simulink model "FINAL_MODEL"  (R2021a)
settings: Solver=VariableStepAuto  StartTime=0.0  StopTime=100  MaxStep=1e-4  RelTol=1e-3
libraries: spsDiodeLib x6, spsIGBTLib x6, spsSeriesRLCBranchLib x3, spsVoltageMeasurementLib x3, spsAsynchronousMachineSIUnitsLib x1, spsDCVoltageSourceLib x1, spsMeanLib x1, pid_lib x1, spspowerguiLib x1
settings Model: Creator=shashank  LastModifiedBy=shashank

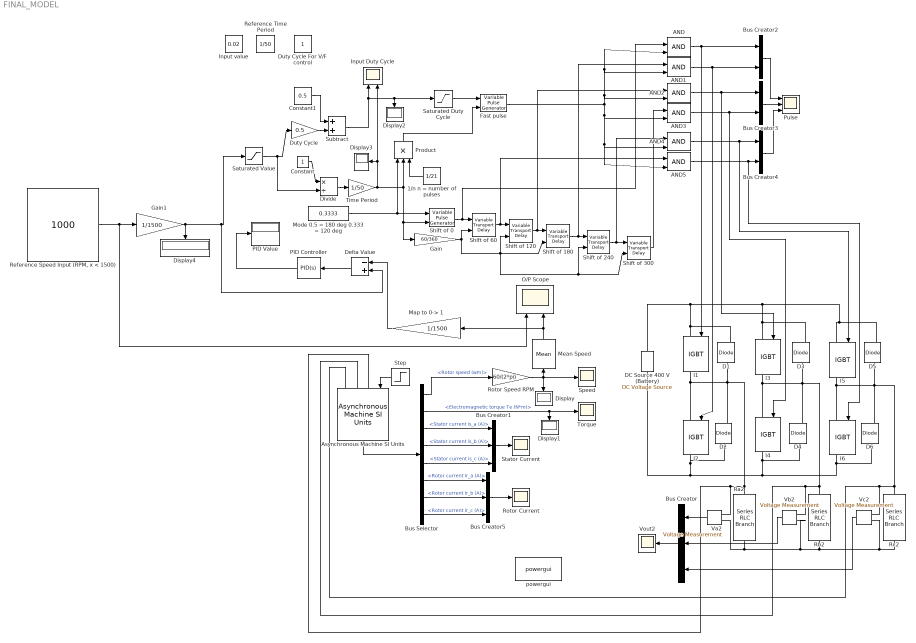
== system FINAL_MODEL ==
  1/n n = number of pulses : Constant  Value=1/21
  AND{,1..5} (6 alike) : Logic  IconShape=distinctive  AllPortsSameDT=off  OutDataTypeStr=boolean
  Asynchronous Machine SI Units : spsAsynchronousMachineSIUnitsLib/Asynchronous Machine SI Units  RotorType=Squirrel-cage  PresetModel="21:  215 HP (160KW) 400 V 50Hz 1487 RPM"  MechanicalLoad=Torque Tm  ShowDetailedParameters=on  ReferenceFrame=Rotor  Units=SI  MeasurementBus=off  NominalParameters=[1.6e+05 400 50]  VoltageRatio=1  Stator=[0.01379 0.000152]  Rotor=[0.007728 0.000152]  Cage1=[0.4155 0.002066]  Cage2=[0.4168 0.0003495]  Lm=0.00769  Mechanical=[2.9 0.05658 2]  PolePairs=2  InitialConditions=[0 0 0 0 0 0 0 0]  SimulateSaturation=off  Saturation=[14.03593122, 27.81365428, 53.79336849, 72.68890987, 97.98006896, 148.6815601, 215.7428561, 302.9841135, 428.7778367 ; 230, 322, 414, 460, 506, 552, 598, 644, 690]  LoadFlowParameters=1492000  TsPowergui=0  TsBlock=-1  IterativeModel=Trapezoidal non iterative  IterativeDiscreteModel=Trapezoidal non iterative  Pmec=1.492e+006
  Bus Creator : BusCreator  Inputs=3
  Bus Creator1 : BusCreator  Inputs=3
  Bus Creator2 : BusCreator  Inputs=2
  Bus Creator3 : BusCreator  Inputs=2
  Bus Creator4 : BusCreator  Inputs=2
  Bus Creator5 : BusCreator  Inputs=3
  Bus Selector : BusSelector  OutputSignals=Mechanical.Rotor speed (wm),Mechanical.Electromagnetic torque Te (N*m),Stator measurements.Stator current is_a (A),Stator measurements.Stator current is_b (A),Stator measurements.Stator current is_c (A),Rotor measurements.Rotor current ir_a (A),Rotor measurements.Rotor current ir_b (A),Rotor measurements.Rotor current ir_c (A)
  Constant : Constant
  Constant1 : Constant  Value=0.5
  D{1..6} (6 alike) : spsDiodeLib/Diode  Ron=0.001  Lon=0  Vf=0.8  IC=0  UseSnubber=0  Rs=500  Cs=250e-9  Measurements=on
  DC Source 400 V (Battery) : spsDCVoltageSourceLib/DC Voltage Source  Amplitude=400  Measurements=None
  Delta Value : Sum  Inputs=-+
  Display{,1..4} (5 alike) : Display
  Divide : Product  Inputs=*/
  Duty Cycle : Gain  Gain=0.5
  Duty Cycle For V/F control : Constant
  Fast pulse : VariablePulseGenerator  SampleTime=0.1
  Gain : Gain  Gain=60/360
  Gain1 : Gain  Gain=1/1500
  I{1..6} (6 alike) : spsIGBTLib/IGBT  Ron=0.001  Lon=0  Vf=1  Tf=1e-6  Tt=2e-6  IC=0  Rs=1e5  Cs=inf  Measurements=on
  Input Duty Cycle : Scope  NumInputPorts=2
  Input value : Constant  Value=0.02
  Map to 0-> 1 : Gain  Gain=1/1500
  Mean Speed : spsMeanLib/Mean  Freq=1  Vinit=0  Ts=0
  Mode 0.5 = 180 deg 0.333 = 120 deg : Constant  Value=0.3333
  O/P Scope : Scope  NumInputPorts=2
  PID Controller : pid_lib/PID Controller  Controller=PID  Form=Parallel  TimeDomain=Continuous-time  UseExternalTs=off  SampleTime=-1  IntegratorMethod=Forward Euler  FilterMethod=Forward Euler  ControllerParametersSource=internal  P=1  I=0.001  D=0  UseFilter=on  N=100  TunerSelectOption=Transfer Function Based (PID Tuner App)  InitialConditionSource=internal  InitialConditionForIntegrator=0  InitialConditionForFilter=0  DifferentiatorICPrevScaledInput=0  ExternalReset=none  TrackingMode=off  Kt=1  LimitOutput=off  SatLimitsSource=internal  UpperSaturationLimit=inf  LowerSaturationLimit=-inf  LinearizeAsGain=on  AntiWindupMode=none  Kb=1  POutMin=[]  POutMax=[]  IOutMin=[]  IOutMax=[]  DOutMin=[]  DOutMax=[]  NOutMin=[]  NOutMax=[]  SumOutMin=[]  SumOutMax=[]  SaturationOutMin=[]  SaturationOutMax=[]  PParamMin=[]  PParamMax=[]  IParamMin=[]  IParamMax=[]  DParamMin=[]  DParamMax=[]  NParamMin=[]  NParamMax=[]  KbParamMin=[]  KbParamMax=[]  KtParamMin=[]  KtParamMax=[]  KbOutMin=[]  KbOutMax=[]  KtOutMin=[]  KtOutMax=[]  IntegratorOutMin=[]  IntegratorOutMax=[]  FilterOutMin=[]  FilterOutMax=[]  SumI1OutMin=[]  SumI1OutMax=[]  SumI2OutMin=[]  SumI2OutMax=[]  SumI3OutMin=[]  SumI3OutMax=[]  SumI4OutMin=[]  SumI4OutMax=[]  SumDOutMin=[]  SumDOutMax=[]  DifferentiatorOutMin=[]  DifferentiatorOutMax=[]  FilterDiffOutCoefMin=[]  FilterDiffOutCoefMax=[]  ReciprocalOutMin=[]  ReciprocalOutMax=[]  SumDenOutMin=[]  SumDenOutMax=[]  SumNumOutMin=[]  SumNumOutMax=[]  DivideOutMin=[]  DivideOutMax=[]  UdiffTsProdOutMin=[]  UdiffTsProdOutMax=[]  NTsProdOutMin=[]  NTsProdOutMax=[]  UintegralTsProdOutMin=[]  UintegralTsProdOutMax=[]  UngainTsProdOutMin=[]  UngainTsProdOutMax=[]  IntegratorContinuousStateAttributes=''  IntegratorStateMustResolveToSignalObject=off  IntegratorRTWStateStorageClass=Auto  FilterContinuousStateAttributes=''  FilterStateMustResolveToSignalObject=off  FilterRTWStateStorageClass=Auto  ParallelPVariant=InternalParameters  IdealPVariant=Disabled  IVariant=InternalParameters  DVariant=InternalParameters  IntegratorVariant=Continuous  SatVariant=Disabled  AWVariant=Passthrough  PCopyVariant=Disabled  TRVariant=Disabled  FdbkBlocksVariant=Forward  IdealPFdbkVariant=Disabled  SatFdbkVariant=Disabled  DerivativeFilterVariant=ContFilter  NVariant=InternalParameters  NCopyVariant=Disabled  FilterICVariant=InternalICsFilter  IntegratorICVariant=InternalICs  ExternalResetVariant=Disabled  TRSumVariant=Passthrough  SumFdbkVariant=Disabled  SumVariant=Sum_PID  TsampFilterVariant=InternalTs  TsampNgainVariant=Passthrough  TsampIntegralVariant=Passthrough  ExternalSaturationOutDataTypeStr=Inherit: Same as second input
  PID Value : Display
  Product : Product  Inputs=3
  Pulse : Scope  NumInputPorts=3
  Ra2 : spsSeriesRLCBranchLib/Series RLC Branch  LConnTagsString=__new0  RConnTagsString=__new0  BranchType=R  Resistance=10  Inductance=1e-3  SetiL0=off  InitialCurrent=0  Capacitance=1e-6  Setx0=off  InitialVoltage=0  Measurements=None
  Rb2 : spsSeriesRLCBranchLib/Series RLC Branch  LConnTagsString=__new0  RConnTagsString=__new0  BranchType=R  Resistance=10  Inductance=1e-3  SetiL0=off  InitialCurrent=0  Capacitance=1e-6  Setx0=off  InitialVoltage=0  Measurements=None
  Rc2 : spsSeriesRLCBranchLib/Series RLC Branch  LConnTagsString=__new0  RConnTagsString=__new0  BranchType=R  Resistance=10  Inductance=1e-3  SetiL0=off  InitialCurrent=0  Capacitance=1e-6  Setx0=off  InitialVoltage=0  Measurements=None
  "Reference Speed Input (RPM, x < 1500)" : Constant  Value=1000
  Reference Time Period : Constant  Value=1/50
  Rotor Current : Scope
  Rotor Speed RPM : Gain  Gain=60/(2*pi)
  Saturated Duty Cycle : Saturate  UpperLimit=1  LowerLimit=0.00000001  LinearizeAsGain=off
  Saturated Value : Saturate  UpperLimit=1  LowerLimit=0.00000001  LinearizeAsGain=off
  Shift of 0 : VariablePulseGenerator  AllowZeroPulseWidth=on  SampleTime=0.1
  Shift of {60,120,180,240,300} (5 alike) : VariableTransportDelay  MaximumDelay=10  FixedBuffer=on  ZeroDelay=on
  Speed : Scope
  Stator Current : Scope
  Step : Step  Time=5  Before=20  After=20  SampleTime=0
  Subtract : Sum
  Time Period : Gain  Gain=1/50
  Torque : Scope
  Va2 : spsVoltageMeasurementLib/Voltage Measurement  PhasorSimulation=off  OutputType=Complex  PSBequivalent=0
  Vb2 : spsVoltageMeasurementLib/Voltage Measurement  PhasorSimulation=off  OutputType=Complex  PSBequivalent=0
  Vc2 : spsVoltageMeasurementLib/Voltage Measurement  PhasorSimulation=off  OutputType=Complex  PSBequivalent=0
  Vout2 : Scope
  powergui : spspowerguiLib/powergui  Priority=1  SimulationMode=Continuous  SampleTime=50e-6  frequency=60  Iterations=50  frequencyindice=0  Pbase=100e6  ErrMax=1e-4  UnitsV=kV  UnitsW=MW  buscounter=0  FunctionMessages=off  echomessages=off  EnableUseOfTLC=off  CurrentSourceSwitches=off  DisableSnubberDevices=off  DisableRonSwitches=off  DisableVfSwitches=off  DisplayEquations=off  AutomaticDiscreteSolvers=off  SolverType=Tustin/Backward Euler (TBE)  Interpol=off  ExternalGateDelay=off  methode=off  Ts=100  x0status=blocks  SPID=on  SwTol=0  HookPort=off  NonlinearTolerance=1e-4  nMaxIteration=100  ContinueOnMaxIteration=off  RestoreLinks=warning  ResistiveCurrentMeasurement=off  Frange=[0:2:500]  Ylog=off  Xlog=on  ShowGrid=off  save=off  variable=ZData  structure=0  ZoomFFT=off  StartTime=0.0  cycles=1  DisplayStyle=1  fundamental=60  FreqAxis=off  MaxFrequency=1000  frequencyindicesteady=1  RmsSteady=1  display=off
  wires:
  Gain/1 -> Shift of 60/2, Shift of 240/2, Shift of 300/2, Shift of 180/2, Shift of 120/2
  Shift of 0/1 -> AND/1, Shift of 60/1
  Mode 0.5 = 180 deg 0.333 = 120 deg/1 -> Shift of 0/1, Product/1
  Time Period/1 -> Product/2, Gain/1, Shift of 0/2, Display3/1, Input Duty Cycle/2
  Shift of 60/1 -> AND5/1, Shift of 120/1
  Shift of 180/1 -> AND1/1, Shift of 240/1
  Shift of 240/1 -> AND4/1, Shift of 300/1
  Shift of 120/1 -> AND2/1, Shift of 180/1
  Bus Creator4/1 -> Pulse/3
  Bus Creator2/1 -> Pulse/1
  Bus Creator3/1 -> Pulse/2
  Subtract/1 -> Saturated Duty Cycle/1, Display2/1, Input Duty Cycle/1
  1/n n = number of pulses/1 -> Product/3
  AND/1 -> I1/1, Bus Creator2/1
  AND1/1 -> I2/1, Bus Creator2/2
  AND3/1 -> I4/1, Bus Creator3/2
  AND2/1 -> Bus Creator3/1, I3/1
  AND4/1 -> Bus Creator4/1, I5/1
  AND5/1 -> I6/1, Bus Creator4/2
  Fast pulse/1 -> AND5/2, AND4/2, AND3/2, AND2/2, AND1/2, AND/2
  Shift of 300/1 -> AND3/1
  Vc2/1 -> Bus Creator/3
  Va2/1 -> Bus Creator/1
  Bus Creator/1 -> Vout2/1
  Vb2/1 -> Bus Creator/2
  Bus Selector/3 -> Bus Creator1/1  "<Stator current is_a (A)>"
  Bus Selector/5 -> Bus Creator1/3  "<Stator current is_c (A)>"
  Bus Selector/7 -> Bus Creator5/2  "<Rotor current ir_b (A)>"
  Rotor Speed RPM/1 -> Speed/1, Display/1, Mean Speed/1
  Bus Creator5/1 -> Rotor Current/1
  Bus Selector/1 -> Rotor Speed RPM/1  "<Rotor speed (wm)>"
  Bus Creator1/1 -> Stator Current/1
  Bus Selector/6 -> Bus Creator5/1  "<Rotor current ir_a (A)>"
  Bus Selector/2 -> Torque/1, Display1/1  "<Electromagnetic torque Te (N*m)>"
  Asynchronous Machine SI Units/1 -> Bus Selector/1
  Step/1 -> Asynchronous Machine SI Units/1
  Bus Selector/8 -> Bus Creator5/3  "<Rotor current ir_c (A)>"
  Bus Selector/4 -> Bus Creator1/2  "<Stator current is_b (A)>"
  Mean Speed/1 -> Map to 0-> 1/1, O/P Scope/2
  Saturated Value/1 -> Duty Cycle/1, Divide/2
  Divide/1 -> Time Period/1
  Constant/1 -> Divide/1
  Duty Cycle/1 -> Subtract/2
  Constant1/1 -> Subtract/1
  Map to 0-> 1/1 -> Delta Value/1
  Gain1/1 -> Delta Value/2, Saturated Value/1, Display4/1
  Delta Value/1 -> PID Controller/1
  PID Controller/1 -> PID Value/1
  Saturated Duty Cycle/1 -> Fast pulse/1
  Product/1 -> Fast pulse/2
  "Reference Speed Input (RPM, x < 1500)"/1 -> O/P Scope/1, Gain1/1
  connections:
  I4/RConn1 -- D6/LConn1 -- I6/RConn1 -- DC Source 400 V (Battery)/LConn1 -- D2/LConn1 -- I2/RConn1 -- D4/LConn1
  I5/RConn1 -- D5/LConn1 -- Vc2/LConn2 -- Asynchronous Machine SI Units/LConn3 -- Rc2/RConn1 -- D6/RConn1 -- I6/LConn1
  Ra2/LConn1 -- Vc2/LConn1 -- Rc2/LConn1 -- Rb2/LConn1 -- Vb2/LConn1 -- Va2/LConn1
  I3/LConn1 -- D5/RConn1 -- I5/LConn1 -- DC Source 400 V (Battery)/RConn1 -- I1/LConn1 -- D1/RConn1 -- D3/RConn1
  I4/LConn1 -- Asynchronous Machine SI Units/LConn2 -- Vb2/LConn2 -- Rb2/RConn1 -- D3/LConn1 -- D4/RConn1 -- I3/RConn1
  D1/LConn1 -- I2/LConn1 -- I1/RConn1 -- Va2/LConn2 -- Asynchronous Machine SI Units/LConn1 -- Ra2/RConn1 -- D2/RConn1
